simulink model "cxema1"  (R2014a)
settings: Solver=ode45  StartTime=0.0  StopTime=50  MaxStep=0.001  MinStep=0.0001  RelTol=1e-3
settings Model: Creator=User  LastModifiedBy=User

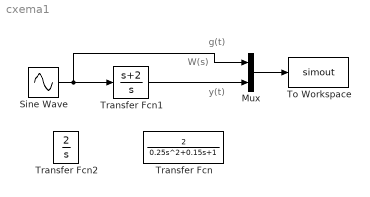
== system cxema1 ==
  note: W(s)
  note: y(t)
  note: g(t)
  Mux : Mux  Inputs=2
  Sine Wave : Sin  Frequency=0.2  SampleTime=0
  To Workspace : ToWorkspace  VariableName=simout  SaveFormat=Timeseries  SampleTime=-1
  Transfer Fcn : TransferFcn  Numerator=[2]  Denominator=[0.25 0.15 1]
  Transfer Fcn1 : TransferFcn  Numerator=[1 2]  Denominator=[1 0]
  Transfer Fcn2 : TransferFcn  Numerator=[2]  Denominator=[1 0]
  wires:
  Mux/1 -> To Workspace/1
  Sine Wave/1 -> Transfer Fcn1/1, Mux/1
  Transfer Fcn1/1 -> Mux/2
